simulink model "Model_Following"  (Simulink 8.4)
settings: Solver=ode45  StartTime=0.0  StopTime=10.0  RelTol=1e-3
values from neighbouring files (symbols this model uses):
  A = [zeros(n) eye(n); Ae Ag]    [AMB_5DOF.m]
  B = [zeros(m); Bi]    [AMB_5DOF.m]
  C = [Ci*inv(T') zeros(5)]    [AMB_5DOF.m]
  Cc = inv(Rc_bar)*B'*inv((A-B*Kc)')*Pc*g    [AMB_5DOF.m]
  Cuc_start = inv(Rc_bar)*(eye(mr) + B'*inv((A-B*Kc)')*Kc')*Rc    [AMB_5DOF.m]
  D = zeros(pr,mr)    [AMB_5DOF.m]
  Ec = -inv(Rc_bar)*((C - D*Kc )*inv( A - B*Kc )*B - D )'*Qc    [AMB_5DOF.m]
  uc_start = [0 0 0 0 0]'    [AMB_5DOF.m]
undefined symbols (not defined in the file or in its folder): Kc, x
settings Model: Creator=koni  LastModifiedBy=123  CovSFcnEnable=on
settings DebuggingCC: FrameProcessingCompatibilityMsg=error

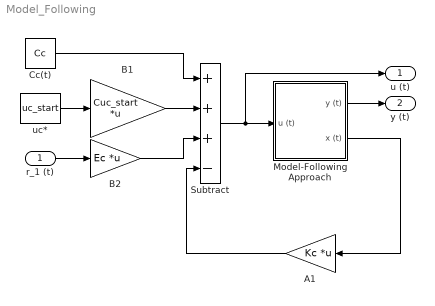
== system Model_Following ==
  r_1 (t) : Inport  PortDimensions=pr
  " Model-Following Approach" : Subsystem
  A1 : Gain  Gain=Kc  Multiplication=Matrix(K*u)
  B1 : Gain  Gain=Cuc_start  Multiplication=Matrix(K*u)
  B2 : Gain  Gain=Ec  Multiplication=Matrix(K*u)
  Cc(t) : Constant  Value=Cc
  Subtract : Sum  Inputs=+++-
  uc* : Constant  Value=uc_start
  u (t) : Outport  PortDimensions=mr
  y (t) : Outport  Port=2  PortDimensions=pr
  wires:
  " Model-Following Approach"/1(y (t)) -> y (t)/1
  Subtract/1 -> " Model-Following Approach"/1(u (t)), u (t)/1
  B2/1 -> Subtract/3
  r_1 (t)/1 -> B2/1
  " Model-Following Approach"/2(x (t)) -> A1/1
  A1/1 -> Subtract/4
  uc*/1 -> B1/1
  B1/1 -> Subtract/2
  Cc(t)/1 -> Subtract/1

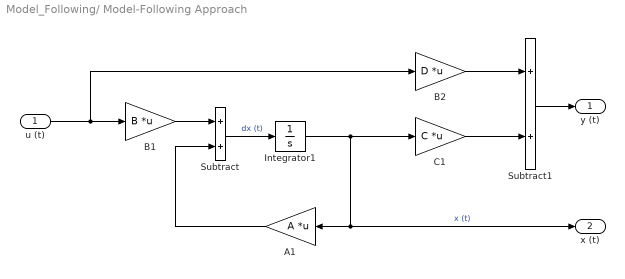
== system Model_Following/ Model-Following Approach ==
  u (t) : Inport  PortDimensions=mr
  A1 : Gain  Gain=A  Multiplication=Matrix(K*u)
  B1 : Gain  Gain=B  Multiplication=Matrix(K*u)
  B2 : Gain  Gain=D  Multiplication=Matrix(K*u)
  C1 : Gain  Gain=C  Multiplication=Matrix(K*u)
  Integrator1 : Integrator  InitialCondition=x(:,1)
  Subtract : Sum
  Subtract1 : Sum
  y (t) : Outport  PortDimensions=pr
  x (t) : Outport  Port=2  PortDimensions=nr
  wires:
  Subtract/1 -> Integrator1/1  "dx (t)"
  Integrator1/1 -> C1/1, A1/1, x (t)/1  "x (t)"
  u (t)/1 -> B1/1, B2/1
  B1/1 -> Subtract/1
  A1/1 -> Subtract/2
  Subtract1/1 -> y (t)/1
  C1/1 -> Subtract1/2
  B2/1 -> Subtract1/1
